simulink model "REAL"  (R2018b)
settings: Solver=VariableStepAuto  StartTime=0.0  StopTime=1000  RelTol=1e-3
values from neighbouring files (symbols this model uses):
  g = 9.8    [param.m]
  k = 1252*1000    (= 1252000)    [param.m]
  M1 = 17*1000    (= 17000)    [param.m]
  M2 = 754.2*1000    (= 754200)    [param.m]
  mu = 0.02    [param.m]
undefined symbols (not defined in the file or in its folder): sigbuilder_block
libraries: simulink x1
settings Model: Creator=pkiop  LastModifiedBy=pkiop

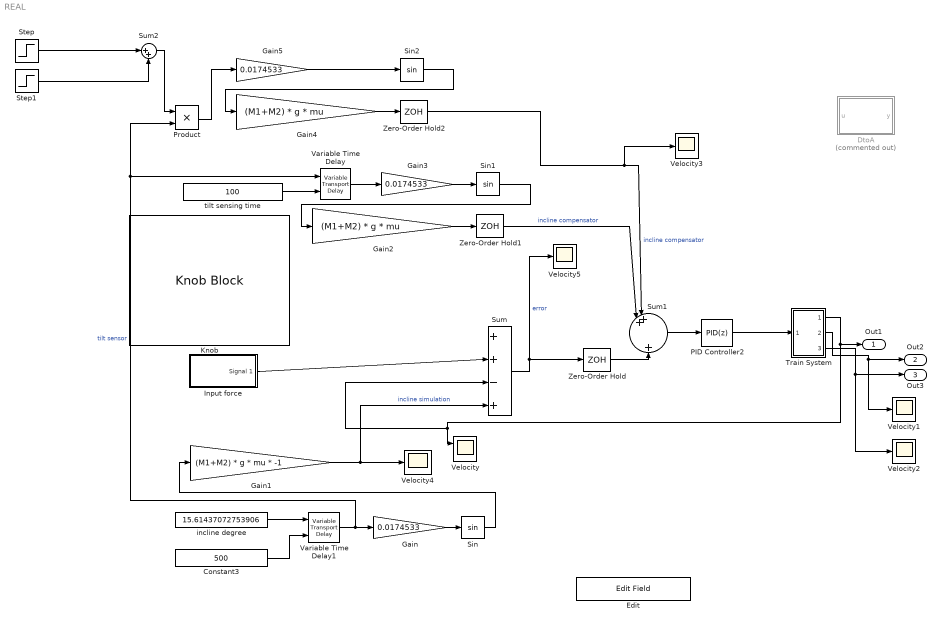
== system REAL ==
  Constant3 : Constant  Value=500
  DtoA : MATLAB Function  Commented=on  TreatAsAtomicUnit=on
  Edit : EditField  WebBlockId=170  LabelPosition=Hide  ShowInitialText=on  Alignment=Center
  Gain : Gain  Gain=0.0174533
  Gain1 : Gain  Gain=(M1+M2) * g * mu * -1
  Gain2 : Gain  Gain=(M1+M2) * g * mu
  Gain3 : Gain  Gain=0.0174533
  Gain4 : Gain  Gain=(M1+M2) * g * mu
  Gain5 : Gain  Gain=0.0174533
  Input force : Subsystem  Tag=STV Subsys  LoadFcn=sigbuilder_block('load');  StartFcn=sigbuilder_block('start');  StopFcn=sigbuilder_block('stop');  ClipboardFcn=sigbuilder_block('clipboard');  mask(Sigbuilder block){tuvar=[0:10]}
      mask help: Simulink:masks:SigbuilderBlock_MD
      mask init:
      | if ~strcmp(get_param(bdroot(gcbh),'SimulationStatus'),'stopped') tuvar = sigbuilder_block('maskInit'); end
      settings: CopyFcn=sigbuilder_block('copy');  DeleteFcn=sigbuilder_block('delete');  ModelCloseFcn=sigbuilder_block('modelClose');  PreSaveFcn=sigbuilder_block('preSave');  PauseFcn=sigbuilder_block('pause');  ContinueFcn=sigbuilder_block('continue');  NameChangeFcn=sigbuilder_block('namechange');  OpenFcn=sigbuilder_block('open',[437.6 199.2 550.4 400 ]);  CloseFcn=sigbuilder_block('close');
      mask Display: plot(0, 0, 100, 100,[2, 2, 32, 32, 2], [68, 8, 8, 68, 68],[32, 2], [38, 38], [32, 19, 2],[53, 60, 44], [32, 17, 17, 2],[16, 16, 31, 31]);txt = getActiveGroup(gcbh);text(2, 100, txt,'verticalAlignment', 'top');
  Knob : KnobBlock  WebBlockId=168  ScaleMin=-30  ScaleMax=30
  PID Controller2 : simulink/Continuous/PID Controller  Controller=PID  Form=Parallel  TimeDomain=Discrete-time  SampleTime=-1  IntegratorMethod=Forward Euler  FilterMethod=Forward Euler  ControllerParametersSource=internal  P=0.01  I=0.08782  D=0  UseFilter=on  N=10  TunerSelectOption=Transfer Function Based (PID Tuner App)  InitialConditionSource=internal  InitialConditionForIntegrator=0  InitialConditionForFilter=0  DifferentiatorICPrevScaledInput=0  ExternalReset=none  TrackingMode=off  Kt=1  LimitOutput=off  UpperSaturationLimit=inf  LowerSaturationLimit=-inf  LinearizeAsGain=on  AntiWindupMode=none  Kb=1  POutMin=[]  POutMax=[]  IOutMin=[]  IOutMax=[]  DOutMin=[]  DOutMax=[]  NOutMin=[]  NOutMax=[]  SumOutMin=[]  SumOutMax=[]  SaturationOutMin=[]  SaturationOutMax=[]  PParamMin=[]  PParamMax=[]  IParamMin=[]  IParamMax=[]  DParamMin=[]  DParamMax=[]  NParamMin=[]  NParamMax=[]  KbParamMin=[]  KbParamMax=[]  KtParamMin=[]  KtParamMax=[]  KbOutMin=[]  KbOutMax=[]  KtOutMin=[]  KtOutMax=[]  IntegratorOutMin=[]  IntegratorOutMax=[]  FilterOutMin=[]  FilterOutMax=[]  SumI1OutMin=[]  SumI1OutMax=[]  SumI2OutMin=[]  SumI2OutMax=[]  SumI3OutMin=[]  SumI3OutMax=[]  SumI4OutMin=[]  SumI4OutMax=[]  SumDOutMin=[]  SumDOutMax=[]  DifferentiatorOutMin=[]  DifferentiatorOutMax=[]  FilterDiffOutCoefMin=[]  FilterDiffOutCoefMax=[]  ReciprocalOutMin=[]  ReciprocalOutMax=[]  SumDenOutMin=[]  SumDenOutMax=[]  SumNumOutMin=[]  SumNumOutMax=[]  DivideOutMin=[]  DivideOutMax=[]  IntegratorContinuousStateAttributes=''  IntegratorStateMustResolveToSignalObject=off  IntegratorRTWStateStorageClass=Auto  FilterContinuousStateAttributes=''  FilterStateMustResolveToSignalObject=off  FilterRTWStateStorageClass=Auto  ParallelPVariant=InternalParameters  IdealPVariant=Disabled  IVariant=InternalParameters  DVariant=InternalParameters  IntegratorVariant=Discrete  SatVariant=Disabled  AWVariant=Passthrough  PCopyVariant=Disabled  TRVariant=Disabled  FdbkBlocksVariant=Forward  IdealPFdbkVariant=Disabled  SatFdbkVariant=Disabled  DerivativeFilterVariant=ForwardEulerFilter  NVariant=InternalParameters  NCopyVariant=Disabled  FilterICVariant=InternalICsFilter  IntegratorICVariant=InternalICs  ExternalResetVariant=Disabled  TRSumVariant=Passthrough  SumFdbkVariant=Disabled  SumVariant=Sum_PID
  Product : Product
  Sin : Trigonometry
  Sin1 : Trigonometry
  Sin2 : Trigonometry
  Step : Step  Time=600  SampleTime=0
  Step1 : Step  Time=700  After=-1  SampleTime=0
  Sum : Sum  Inputs=|+|+-|+
  Sum1 : Sum  Inputs=|++||||||+
  Sum2 : Sum  Inputs=|++
  "Train System " : Subsystem
  Variable Time Delay : VariableTransportDelay  MaximumDelay=9999
  Variable Time Delay1 : VariableTransportDelay  MaximumDelay=9999
  Velocity : Scope  NumInputPorts=2
  Velocity{1..5} (5 alike) : Scope
  Zero-Order Hold : ZeroOrderHold  SampleTime=0.1
  Zero-Order Hold1 : ZeroOrderHold  SampleTime=0.1
  Zero-Order Hold2 : ZeroOrderHold  SampleTime=0.1
  incline degree : Constant  Value=15.61437072753906
  tilt sensing time : Constant  Value=100
  Out1 : Outport
  Out2 : Outport  Port=2
  Out3 : Outport  Port=3
  wires:
  "Train System "/2(Out2) -> Velocity1/1, Out2/1
  "Train System "/3(Out3) -> Velocity2/1, Out3/1
  "Train System "/1(Out1) -> Out1/1, Velocity/1, Sum/3
  Sum/1 -> Zero-Order Hold/1, Velocity5/1  "error"
  Gain1/1 -> Sum/4, Velocity4/1  "incline simulation"
  Gain/1 -> Sin/1
  Sin/1 -> Gain1/1
  Gain3/1 -> Sin1/1
  Gain2/1 -> Zero-Order Hold1/1
  Sum1/1 -> PID Controller2/1
  Variable Time Delay1/1 -> Variable Time Delay/1, Product/2, Gain/1  "tilt sensor"
  Variable Time Delay/1 -> Gain3/1
  tilt sensing time/1 -> Variable Time Delay/2
  incline degree/1 -> Variable Time Delay1/1
  Sin1/1 -> Gain2/1
  Constant3/1 -> Variable Time Delay1/2
  Input force/1(Signal 1) -> Sum/2
  PID Controller2/1 -> "Train System "/1(In1)
  Gain4/1 -> Zero-Order Hold2/1
  Sin2/1 -> Gain4/1
  Zero-Order Hold2/1 -> Velocity3/1, Sum1/1  "incline compensator"
  Gain5/1 -> Sin2/1
  Zero-Order Hold/1 -> Sum1/3
  Zero-Order Hold1/1 -> Sum1/2  "incline compensator"
  Step/1 -> Sum2/1
  Step1/1 -> Sum2/2
  Sum2/1 -> Product/1
  Product/1 -> Gain5/1

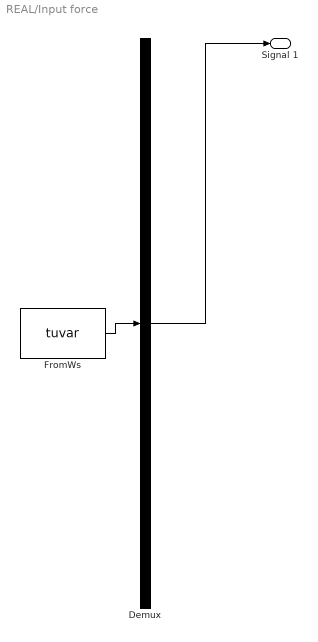
== system REAL/Input force ==
  Demux : Demux  Tag=STV Demux  Outputs=1
  FromWs : FromWorkspace  Tag=STV FromWs  VariableName=tuvar  SampleTime=0
      SigBuilderData=|
      | common.afterFinalStr = 'Extrapolate'
      | common.sampleTime = 0
      | dataSet.timeRange = [0 800]
      | dataSet.name = 'Group 1'
      | sbobj.Groups.Name = 'Group 1'
      | sbobj.Groups.Signals.Name = 'Signal 1'
      | sbobj.Groups.Signals.XData = [0 1.26 1.26 360 360 800]
      | sbobj.Groups.Signals.YData = [0 0 384000 384000 0 0]
      | sbobj.Groups.TimeRange = [0 800]
  Signal 1 : Outport  Tag=STV Outport
  wires:
  Demux/1 -> Signal 1/1
  FromWs/1 -> Demux/1

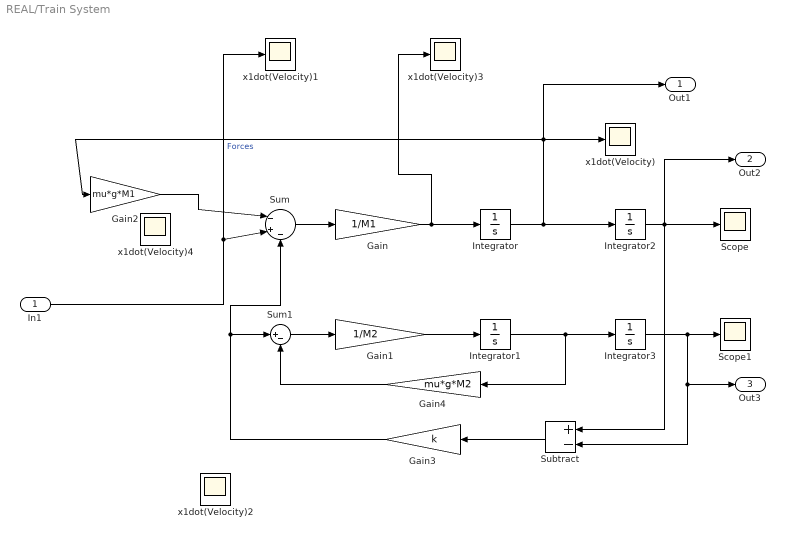
== system REAL/Train System  ==
  In1 : Inport
  Gain : Gain  Gain=1/M1
  Gain1 : Gain  Gain=1/M2
  Gain2 : Gain  Gain=mu*g*M1
  Gain3 : Gain  Gain=k
  Gain4 : Gain  Gain=mu*g*M2
  Integrator{,1..3} (4 alike) : Integrator
  Scope : Scope
  Scope1 : Scope
  Subtract : Sum  Inputs=+-
  Sum : Sum  Inputs=|-+-
  Sum1 : Sum  Inputs=|+-
  x1dot(Velocity){,1..4} (5 alike) : Scope
  Out1 : Outport
  Out2 : Outport  Port=2
  Out3 : Outport  Port=3
  wires:
  Integrator3/1 -> Out3/1, Subtract/2, Scope1/1
  Integrator2/1 -> Out2/1, Subtract/1, Scope/1
  Gain/1 -> x1dot(Velocity)3/1, Integrator/1
  Integrator/1 -> Out1/1, Gain2/1, x1dot(Velocity)/1, Integrator2/1
  Gain1/1 -> Integrator1/1
  Integrator1/1 -> Gain4/1, Integrator3/1
  Sum1/1 -> Gain1/1
  In1/1 -> x1dot(Velocity)1/1, Sum/2  "Forces"
  Subtract/1 -> Gain3/1
  Gain3/1 -> Sum/3, Sum1/1
  Gain4/1 -> Sum1/2
  Sum/1 -> Gain/1
  Gain2/1 -> Sum/1

== matlab function REAL/DtoA ==
  data: u input; y output
function y = fcn(u)
y = d2c(u,'method')
